simulink model "EVTOL_6DOF_Plant_V2"  (R2025b)
settings: Solver=VariableStepAuto  StartTime=0.0  StopTime=10.0  RelTol=1e-3
undefined symbols (not defined in the file): avlAero, eul_init, F, g, J, Light, magnitude, Mass, MIL, omega_init, pos_init, rho, use_avl_aero, V_init
libraries: Flight_Controls_lib x13, simulink_extras x4, aerolibwind2 x1
settings Model: Creator=zbrown  LastModifiedBy=ryanc

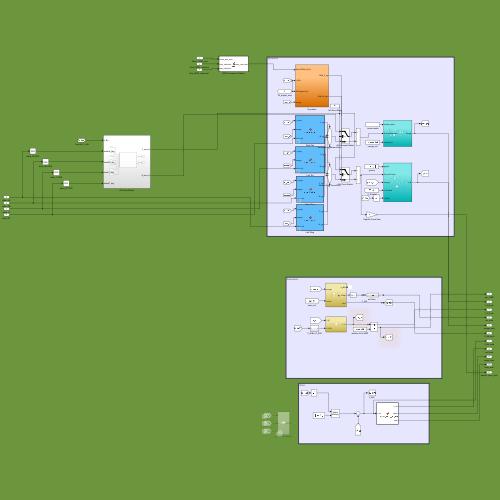
[thumbnail: Simulink's stored preview of the top-level diagram]
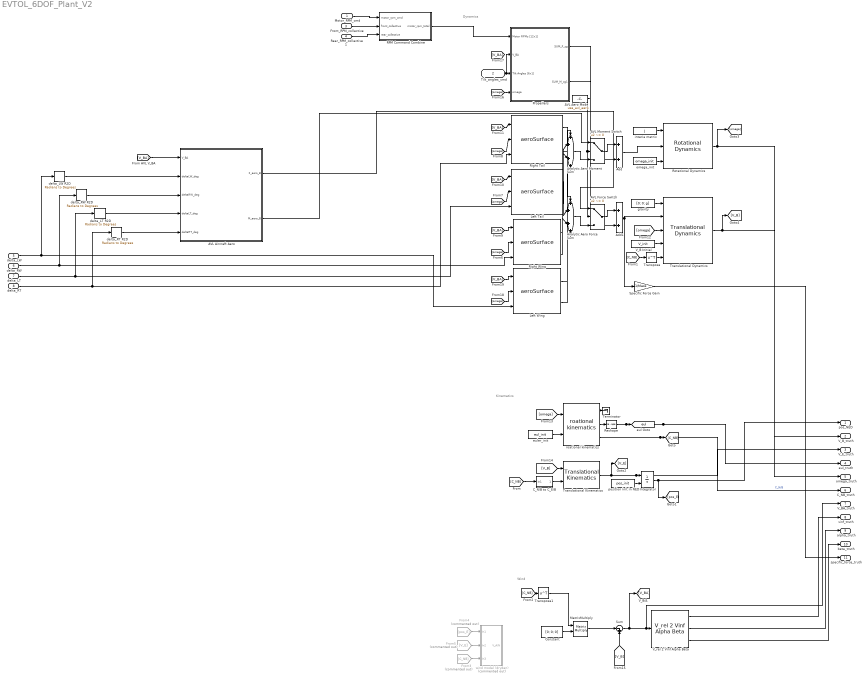
== system EVTOL_6DOF_Plant_V2 ==
  note: Wind
  note: Dynamics
  note: Kinematics
  Motor_RPM_cmd : Inport  PortDimensions=12
  Tilt_angles_cmd : Inport  Port=2  PortDimensions=6
  Front_RPM_collective : Inport  Port=3
  Rear_RPM_collective1 : Inport  Port=4
  delta_LW : Inport  Port=5
  delta_RW : Inport  Port=6
  delta_LT : Inport  Port=7
  delta_RT : Inport  Port=8
  " V_B Initial" : Constant  Value=V_init
  " gravity" : Constant  Value=[0; 0; g]
  " interia matrix" : Constant  Value=J
  AVL Aero Mode : Constant  Value=use_avl_aero
  AVL Aircraft Aero : Subsystem
  AVL Force Switch : Switch  Criteria=u2 ~= 0  Threshold=0.5  SaturateOnIntegerOverflow=off  InputSameDT=off
  AVL Moment Switch : Switch  Criteria=u2 ~= 0  Threshold=0.5  SaturateOnIntegerOverflow=off  InputSameDT=off
  Add : Sum
  Add1 : Sum
  Analytic Aero Force Sum : Sum  Inputs=++++
  Analytic Aero Moment Sum : Sum  Inputs=++++
  C_N/B to C_E/B : Subsystem
  Constant : Constant  Value=[0; 0; 0]
  From3 : From  Commented=on  GotoTag=C_NB
  From4 : From  Commented=on  GotoTag=pos_E
  From5 : From  Commented=on  GotoTag=V_E
  Integrator : Integrator  InitialConditionSource=external
  Left Tail : Flight_Controls_lib/aeroSurface  surf=tailL  CG=CG
  Left Wing : Flight_Controls_lib/aeroSurface  surf=wingL  CG=CG
  MatrixMultiply : Product  Multiplication=Matrix(*)
  Propellers : Subsystem
  RPM Command Combine : MATLAB Function  TreatAsAtomicUnit=on
  Reshape : Reshape
  Right Tail : Flight_Controls_lib/aeroSurface  surf=tailR  CG=CG
  Right Wing : Flight_Controls_lib/aeroSurface  surf=wingR  CG=CG
  Rotational Dynamics : Flight_Controls_lib/Rotational Dynamics  SystemSampleTime=-1  VariantActivationTime=update diagram  EmptyChoice=off  PassThrough=off  PassThroughVariantControl=(default)  EmptyChoiceVariantControl=(default)  AllowFlexibleInterface=on  Latency=0  AutoFrameSizeCalculation=off
  Specific Force Gain : Gain  Gain=1/Mass
  Sum : Sum  Inputs=|-+
  Terminator : Terminator
  Translational Dynamics : Flight_Controls_lib/Translational Dynamics  SystemSampleTime=-1  VariantActivationTime=update diagram  EmptyChoice=off  PassThrough=off  PassThroughVariantControl=(default)  EmptyChoiceVariantControl=(default)  AllowFlexibleInterface=on  Latency=0  AutoFrameSizeCalculation=off
  Translational Kinematics : Flight_Controls_lib/Translational Kinematics  SystemSampleTime=-1  VariantActivationTime=update diagram  EmptyChoice=off  PassThrough=off  PassThroughVariantControl=(default)  EmptyChoiceVariantControl=(default)  AllowFlexibleInterface=on  Latency=0  AutoFrameSizeCalculation=off
  Transpose : Math  Operator=transpose
  Transpose1 : Math  Operator=transpose
  V_rel 2 Vinf Alpha Beta : Flight_Controls_lib/V_rel 2 Vinf Alpha Beta  SystemSampleTime=-1  VariantActivationTime=update diagram  EmptyChoice=off  PassThrough=off  PassThroughVariantControl=(default)  EmptyChoiceVariantControl=(default)  AllowFlexibleInterface=on  Latency=0  AutoFrameSizeCalculation=off
  delta_LT R2D : simulink_extras/Transformations/Radians to Degrees
  delta_LW R2D : simulink_extras/Transformations/Radians to Degrees
  delta_RT R2D : simulink_extras/Transformations/Radians to Degrees
  delta_RW R2D : simulink_extras/Transformations/Radians to Degrees
  euler_init : Constant  Value=eul_init
  omega_init : Constant  Value=omega_init
  position init in NED : Constant  Value=pos_init
  roational kinematics : Flight_Controls_lib/roational kinematics  SystemSampleTime=-1  VariantActivationTime=update diagram  EmptyChoice=off  PassThrough=off  PassThroughVariantControl=(default)  EmptyChoiceVariantControl=(default)  AllowFlexibleInterface=on  Latency=0  AutoFrameSizeCalculation=off
  wind model (dryden) : Subsystem  Commented=on
  pos_NED : Outport
  V_B_truth : Outport  Port=2
  V_E_truth : Outport  Port=3
  eul_truth : Outport  Port=4
  omega_truth : Outport  Port=5
  C_NB_truth : Outport  Port=6
  V_BA_truth : Outport  Port=7
  vinf_truth : Outport  Port=8
  alpha_truth : Outport  Port=9
  beta_truth : Outport  Port=10
  specific_force_truth : Outport  Port=11
  tag scope: eul=global
  wires:
  Transpose/1 -> Translational Dynamics/5
  roational kinematics/3 -> [C_NB], C_NB_truth/1  "C_N/B"
  roational kinematics/1 -> Terminator/1
  roational kinematics/2 -> Reshape/1
  Rotational Dynamics/1 -> omega_truth/1, [omega]
  Translational Dynamics/1 -> V_B_truth/1, [V_B]
  Translational Kinematics/1 -> V_E_truth/1, Integrator/1, [V_E]
  position init in NED/1 -> Integrator/2
  Integrator/1 -> pos_NED/1, [pos_E]
  euler_init/1 -> roational kinematics/2
  omega_init/1 -> Rotational Dynamics/3
  Add/1 -> Rotational Dynamics/2
  " interia matrix"/1 -> Rotational Dynamics/1
  " gravity"/1 -> Translational Dynamics/1
  Add1/1 -> Translational Dynamics/2, Specific Force Gain/1
  " V_B Initial"/1 -> Translational Dynamics/4
  Reshape/1 -> eul_truth/1, [eul]
  C_N/B to C_E/B/1(Out1) -> Translational Kinematics/2
  [C_NB] -> C_N/B to C_E/B/1(In1)
  [C_NB] -> Transpose/1
  MatrixMultiply/1 -> Sum/1
  Transpose1/1 -> MatrixMultiply/1
  [C_NB] -> Transpose1/1
  Sum/1 -> V_BA_truth/1, V_rel 2 Vinf Alpha Beta/1, [V_BA]
  From4/1 -> wind model (dryden)/1(In1)
  From5/1 -> wind model (dryden)/2(In2)
  From3/1 -> wind model (dryden)/3(In3)
  [omega] -> Right Wing/2
  [omega] -> Left Tail/2
  [V_BA] -> Right Wing/1
  [V_BA] -> Left Tail/1
  [V_BA] -> Right Tail/1
  V_rel 2 Vinf Alpha Beta/1 -> vinf_truth/1
  V_rel 2 Vinf Alpha Beta/2 -> alpha_truth/1
  V_rel 2 Vinf Alpha Beta/3 -> beta_truth/1
  [omega] -> Translational Dynamics/3
  [omega] -> roational kinematics/1
  [V_B] -> Translational Kinematics/1
  Right Wing/1 -> Analytic Aero Force Sum/3
  Left Tail/1 -> Analytic Aero Force Sum/2
  Right Tail/1 -> Analytic Aero Force Sum/1
  Right Tail/2 -> Analytic Aero Moment Sum/1
  Left Tail/2 -> Analytic Aero Moment Sum/2
  Right Wing/2 -> Analytic Aero Moment Sum/3
  [V_B] -> Sum/2
  [omega] -> Right Tail/2
  Tilt_angles_cmd/1 -> Propellers/3(Tilt Angles [6x1]), Propellers/2(V_BA)
  [omega] -> Propellers/4(omega)
  Propellers/1(SUM_F_cg) -> Add/2
  Propellers/2(SUM_M_cg1) -> Add1/2
  [omega] -> Left Wing/2
  [V_BA] -> Left Wing/1
  Left Wing/2 -> Analytic Aero Moment Sum/4
  Left Wing/1 -> Analytic Aero Force Sum/4
  [V_BA] -> AVL Aircraft Aero/1(V_BA)
  Analytic Aero Force Sum/1 -> AVL Force Switch/3
  AVL Aero Mode/1 -> AVL Force Switch/2, AVL Moment Switch/2
  AVL Aircraft Aero/1(F_aero_B) -> AVL Force Switch/1
  Analytic Aero Moment Sum/1 -> AVL Moment Switch/3
  AVL Aircraft Aero/2(M_aero_B) -> AVL Moment Switch/1
  AVL Force Switch/1 -> Add1/1
  AVL Moment Switch/1 -> Add/1
  Constant/1 -> MatrixMultiply/2
  delta_LW/1 -> Left Wing/3, delta_LW R2D/1
  delta_RW/1 -> delta_RW R2D/1, Right Wing/3
  delta_LT/1 -> delta_LT R2D/1, Left Tail/3
  delta_RT/1 -> delta_RT R2D/1, Right Tail/3
  delta_LW R2D/1 -> AVL Aircraft Aero/2(deltaLW_deg)
  delta_RW R2D/1 -> AVL Aircraft Aero/3(deltaRW_deg)
  delta_LT R2D/1 -> AVL Aircraft Aero/4(deltaLT_deg)
  delta_RT R2D/1 -> AVL Aircraft Aero/5(deltaRT_deg)
  Motor_RPM_cmd/1 -> RPM Command Combine/1(motor_rpm_cmd)
  Front_RPM_collective/1 -> RPM Command Combine/2(front_collective)
  Rear_RPM_collective1/1 -> RPM Command Combine/3(rear_collective)
  RPM Command Combine/1(motor_rpm_total) -> Propellers/1(Motor RPMs [12x1])
  Specific Force Gain/1 -> specific_force_truth/1

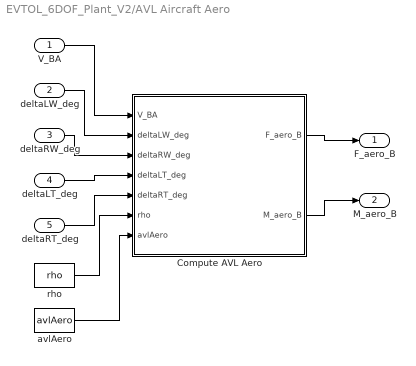
== system EVTOL_6DOF_Plant_V2/AVL Aircraft Aero ==
  V_BA : Inport
  deltaLW_deg : Inport  Port=2
  deltaRW_deg : Inport  Port=3
  deltaLT_deg : Inport  Port=4
  deltaRT_deg : Inport  Port=5
  Compute AVL Aero : MATLAB Function  TreatAsAtomicUnit=on
  avlAero : Constant  Value=avlAero  OutDataTypeStr=Bus: avlAeroBus
  rho : Constant  Value=rho
  F_aero_B : Outport
  M_aero_B : Outport  Port=2
  wires:
  V_BA/1 -> Compute AVL Aero/1(V_BA)
  deltaLW_deg/1 -> Compute AVL Aero/2(deltaLW_deg)
  deltaRW_deg/1 -> Compute AVL Aero/3(deltaRW_deg)
  deltaLT_deg/1 -> Compute AVL Aero/4(deltaLT_deg)
  deltaRT_deg/1 -> Compute AVL Aero/5(deltaRT_deg)
  rho/1 -> Compute AVL Aero/6(rho)
  avlAero/1 -> Compute AVL Aero/7(avlAero)
  Compute AVL Aero/1(F_aero_B) -> F_aero_B/1
  Compute AVL Aero/2(M_aero_B) -> M_aero_B/1

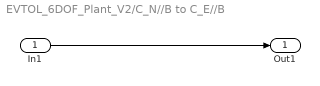
== system EVTOL_6DOF_Plant_V2/C_N//B to C_E//B ==
  In1 : Inport
  Out1 : Outport
  wires:
  In1/1 -> Out1/1

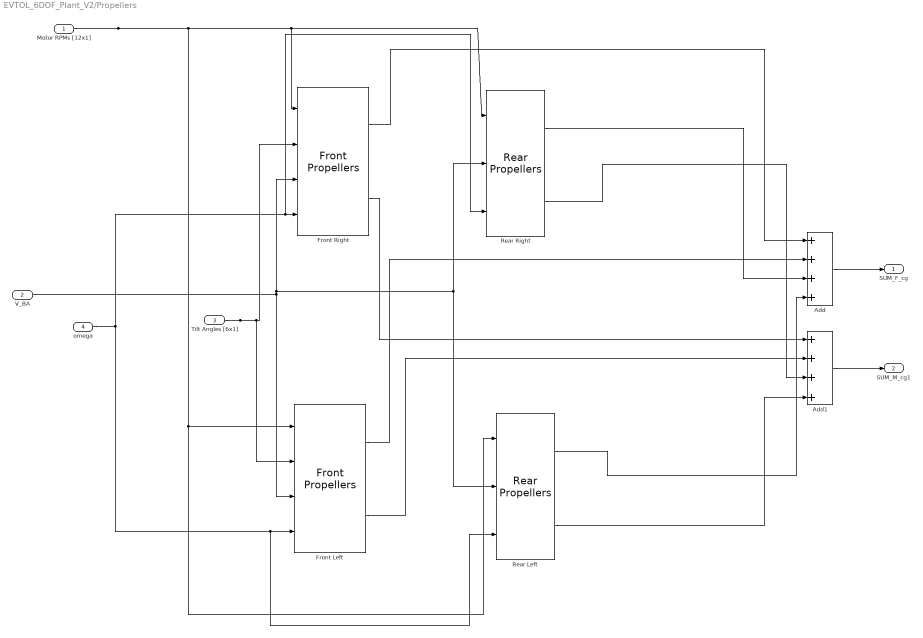
== system EVTOL_6DOF_Plant_V2/Propellers ==
  Motor RPMs [12x1] : Inport
  V_BA : Inport  Port=2
  Tilt Angles [6x1] : Inport  Port=3
  omega : Inport  Port=4
  Add : Sum  Inputs=++++
  Add1 : Sum  Inputs=++++
  Front Left : Flight_Controls_lib/Front Propellers  pivot_pos=prop.posFL  hub_offset=prop.hub_offset  kT=prop.k_Thrust  kQ=prop.k_Torque  CG=CG  spin_dir=prop.Lspin_dir
  Front Right : Flight_Controls_lib/Front Propellers  pivot_pos=prop.posFR  hub_offset=prop.hub_offset  kT=prop.k_Thrust  kQ=prop.k_Torque  CG=CG  spin_dir=prop.Rspin_dir
  Rear Left : Flight_Controls_lib/Rear Propellers  prop_pos=prop.posRL  kT=prop.k_Thrust  kQ=prop.k_Torque  CG=CG  spin_dir=prop.Lspin_dir
  Rear Right : Flight_Controls_lib/Rear Propellers  prop_pos=prop.posRR  kT=prop.k_Thrust  kQ=prop.k_Torque  CG=CG  spin_dir=prop.Rspin_dir
  SUM_F_cg : Outport
  SUM_M_cg1 : Outport  Port=2
  wires:
  V_BA/1 -> Front Right/3, Rear Left/2, Rear Right/2, Front Left/3
  Add/1 -> SUM_F_cg/1
  Add1/1 -> SUM_M_cg1/1
  Motor RPMs [12x1]/1 -> Front Left/1, Rear Left/1, Front Right/1, Rear Right/1
  Tilt Angles [6x1]/1 -> Front Right/2, Front Left/2
  omega/1 -> Rear Right/3, Front Right/4, Rear Left/3, Front Left/4
  Front Right/1 -> Add/1
  Rear Right/1 -> Add/3
  Front Left/1 -> Add/2
  Rear Left/1 -> Add/4
  Front Right/2 -> Add1/1
  Rear Right/2 -> Add1/3
  Front Left/2 -> Add1/2
  Rear Left/2 -> Add1/4

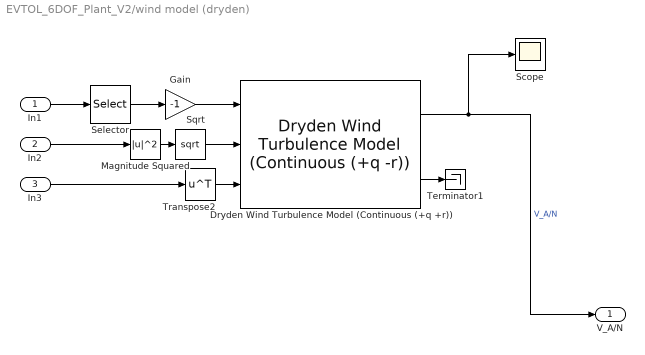
== system EVTOL_6DOF_Plant_V2/wind model (dryden) ==
  In1 : Inport
  In2 : Inport  Port=2
  In3 : Inport  Port=3
  Dryden Wind Turbulence Model (Continuous (+q +r)) : aerolibwind2/Dryden Wind Turbulence Model  (Continuous (+q -r))  units=Metric (MKS)  spec=MIL-F-8785C  model=Continuous Dryden (+q +r)  W20=15  Wdeg=0  TurbProb=10^-2 - Light  L_high=533.4  Wingspan=10  ts=0.1  Seed=[23341 23342 23343 23344]  T_on=on
      settings: LibrarySourceBlock=|
      | aerolibwind2/Dryden Wind Turbulence Model
      | (Continuous (+q +r))
  Gain : Gain  Gain=-1
  Magnitude Squared : Math  Operator=magnitude^2
  Scope : Scope
  Selector : Selector  InputPortWidth=3  IndexOptions=Index vector (dialog)  Indices=[3]  OutputSizes=1
  Sqrt : Sqrt
  Terminator1 : Terminator
  Transpose2 : Math  Operator=transpose
  V_A/N : Outport
  wires:
  In1/1 -> Selector/1
  Sqrt/1 -> Dryden Wind Turbulence Model (Continuous (+q +r))/2
  Dryden Wind Turbulence Model (Continuous (+q +r))/1 -> V_A/N/1, Scope/1  "V_A/N"
  In3/1 -> Transpose2/1
  Transpose2/1 -> Dryden Wind Turbulence Model (Continuous (+q +r))/3
  In2/1 -> Magnitude Squared/1
  Dryden Wind Turbulence Model (Continuous (+q +r))/2 -> Terminator1/1
  Gain/1 -> Dryden Wind Turbulence Model (Continuous (+q +r))/1
  Selector/1 -> Gain/1
  Magnitude Squared/1 -> Sqrt/1

== matlab function EVTOL_6DOF_Plant_V2/AVL Aircraft Aero/Compute AVL Aero ==
  data: V_BA input; F_aero_B output; deltaLW_deg input; deltaRW_deg input; deltaLT_deg input; deltaRT_deg input; rho input; avlAero input; M_aero_B output
function [F_aero_B, M_aero_B] = fcn(V_BA, deltaLW_deg, deltaRW_deg, deltaLT_deg, deltaRT_deg, rho, avlAero)
%#codegen
[F_aero_B, M_aero_B] = avl_aircraft_aero_eval(V_BA, deltaLW_deg, deltaRW_deg, deltaLT_deg, deltaRT_deg, rho, avlAero);
end

== matlab function EVTOL_6DOF_Plant_V2/RPM Command Combine ==
  data: motor_rpm_cmd input; motor_rpm_total output; front_collective input; rear_collective input
function motor_rpm_total = fcn(motor_rpm_cmd, front_collective, rear_collective)

motor_rpm_total = motor_rpm_cmd(:);
if numel(motor_rpm_total) ~= 12
    motor_rpm_total = zeros(12, 1);
end
motor_rpm_total(1:6) = motor_rpm_total(1:6) + front_collective;
motor_rpm_total(7:12) = motor_rpm_total(7:12) + rear_collective;
end
